simulink model "rollangleacc"  (R2020a)
settings: Solver=VariableStepAuto  StartTime=0.0  StopTime=10.0  RelTol=1e-3
undefined symbols (not defined in the file): I, Ixx, Iyy, Izz, Jr
settings Model: Creator=Muni Kumar  LastModifiedBy=Muni Kumar

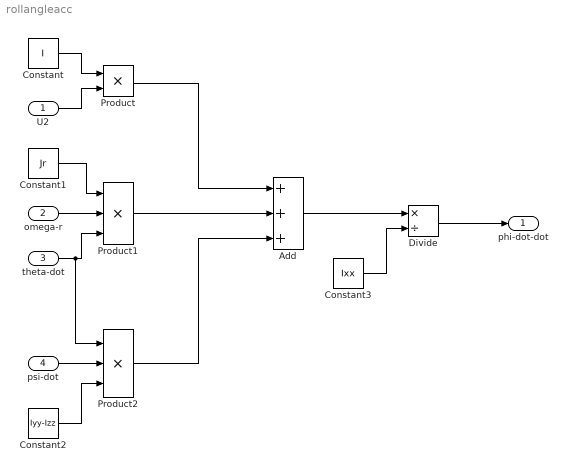
== system rollangleacc ==
  U2 : Inport
  omega-r : Inport  Port=2
  theta-dot : Inport  Port=3
  psi-dot : Inport  Port=4
  Add : Sum  Inputs=+++
  Constant : Constant  Value=I
  Constant1 : Constant  Value=Jr
  Constant2 : Constant  Value=Iyy-Izz
  Constant3 : Constant  Value=Ixx
  Divide : Product  Inputs=*/
  Product : Product
  Product1 : Product  Inputs=3
  Product2 : Product  Inputs=3
  phi-dot-dot : Outport
  wires:
  Constant/1 -> Product/1
  U2/1 -> Product/2
  Constant1/1 -> Product1/1
  omega-r/1 -> Product1/2
  theta-dot/1 -> Product2/1, Product1/3
  psi-dot/1 -> Product2/2
  Constant2/1 -> Product2/3
  Product1/1 -> Add/2
  Product/1 -> Add/1
  Product2/1 -> Add/3
  Add/1 -> Divide/1
  Constant3/1 -> Divide/2
  Divide/1 -> phi-dot-dot/1
